simulink model "FFT_acquisition"  (R2022a)
settings: Solver=VariableStepAuto  StartTime=0.0  StopTime=0.001  RelTol=1e-3
values from neighbouring files (symbols this model uses):
  v = 2.5    [test.m]    (also in test_Datacode.m = 5)
undefined symbols (not defined in the file or in its folder): fdesignblkfcn, gcbh
libraries: simulink x3, dspxfrm3 x3, commchan3 x1, dsparch4 x1, dspfdesign x1, commrandsrc3 x1
settings Model: Creator=sky 2020  LastModifiedBy=sky 2020

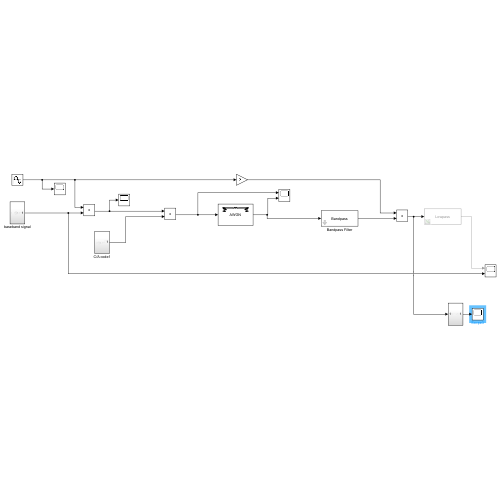
[thumbnail: Simulink's stored preview of the top-level diagram]
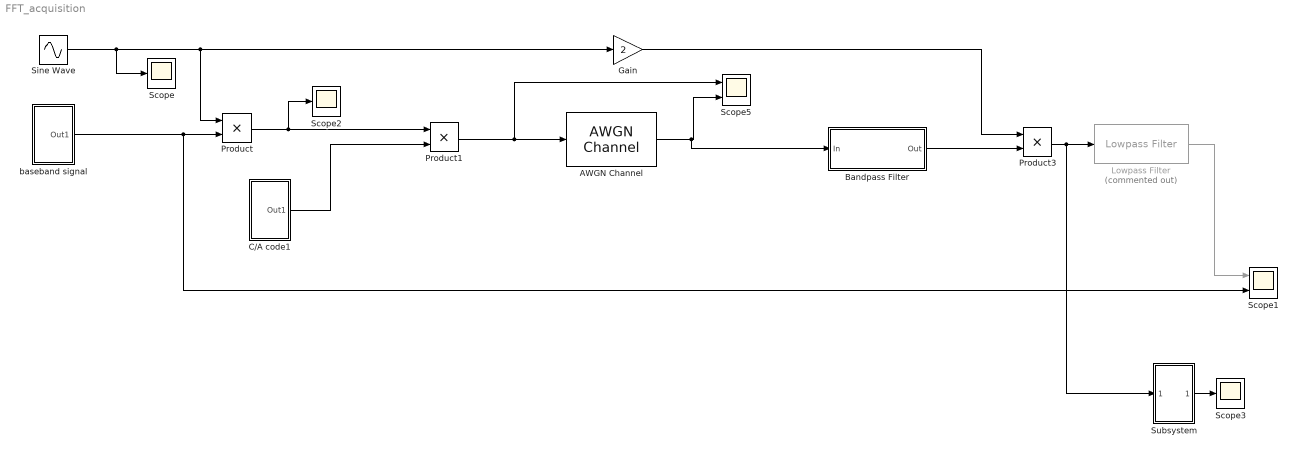
== system FFT_acquisition ==
  AWGN Channel : commchan3/AWGN Channel  InputProcessing=Columns as channels (frame based)  seed=67  noiseMode="Signal to noise ratio  (SNR)"  EbNodB=0  EsNodB=10  SNRdB=0  bitsPerSym=1  Ps=1  Tsym=1  variance=1
  Bandpass Filter : Subsystem  DialogController=fdesignblkfcn  InitFcn=fdesignblkfcn(gcbh, {'InitFcn'});  mask(Bandpass Filter){}
      mask help: Design a bandpass filter
      settings: CopyFcn=fdesignblkfcn(gcbh, {'CopyFcn'});
      mask Help: helpview(mapfilelocation('dsp'), 'dspbandpassfilter');
      mask Display: disp('Bandpass');
  C/A code1 : Subsystem
  Gain : Gain  Gain=2
  Lowpass Filter : dspfdesign/Lowpass Filter  Commented=on  FilterType=FIR  DesignForMinimumOrder=on  FilterOrder=50  PassbandFrequency=1.2e3  StopbandFrequency=2e3  PassbandRipple=0.1  StopbandAttenuation=60  InheritSampleRate=off  SampleRate=157.742e2  SimulateUsing=Interpreted execution  roundingMode=Floor  coeffsDataTypeStr=fixdt(1,16)
  Product : Product
  Product1 : Product
  Product3 : Product
  Scope : Scope
  Scope1 : Scope  NumInputPorts=2
  Scope2 : Scope
  Scope3 : Scope
  Scope5 : Scope  NumInputPorts=2
  Sine Wave : Sin  Frequency=2*pi*157.542e6  Phase=pi/2  SampleTime=1/(v*157.542e6)
  Subsystem : Subsystem
  baseband signal : Subsystem
  wires:
  Sine Wave/1 -> Scope/1, Gain/1, Product/1
  AWGN Channel/1 -> Bandpass Filter/1(In), Scope5/2
  Lowpass Filter/1 -> Scope1/1
  Bandpass Filter/1(Out) -> Product3/2
  Product1/1 -> Scope5/1, AWGN Channel/1
  baseband signal/1(Out1) -> Scope1/2, Product/2
  C/A code1/1(Out1) -> Product1/2
  Gain/1 -> Product3/1
  Product/1 -> Scope2/1, Product1/1
  Product3/1 -> Subsystem/1(In1), Lowpass Filter/1
  Subsystem/1(Out1) -> Scope3/1

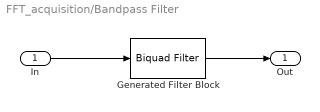
== system FFT_acquisition/Bandpass Filter ==
  In : Inport
  Generated Filter Block : dsparch4/Biquad Filter  Tag=BlockMethodSubSystem  FilterSource=Dialog parameters  CoeffSource=Specify via dialog  FilterObject=BQF  IIRFiltStruct=Direct form II  BiQuadCoeffs=[0.00380302990539071279 0 -0.00380302990539071279 1 1.61904346999335025 0.998458791755205466;0.00222628283797649028 0 -0.00222628283797649028 1 1.61451631506587345 0.998450612907040735;0.851459124863951367 0 -0.851459124863951367 1 1.61553762151329305 0.996911779330365899]  ScaleValues=[0.000919689030413472098;1;1;1]  IC=0  ICnum=0  ICden=0  a0Flag=Warning  optimizeScaleValues=off  ScaleValueMode=Specify via input port (g)  InputProcessing=Columns as channels (frame based)  roundingMode=Floor  overflowMode=off  scaleValueFracLength=14  denProdOutputFracLength=30  denAccumFracLength=30  secondMemoryFracLength=15
  Out : Outport  VectorParamsAs1DForOutWhenUnconnected=off
  wires:
  In/1 -> Generated Filter Block/1
  Generated Filter Block/1 -> Out/1

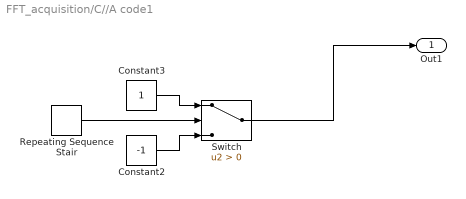
== system FFT_acquisition/C//A code1 ==
  Constant2 : Constant  Value=-1
  Constant3 : Constant
  Repeating Sequence Stair : simulink/Sources/Repeating Sequence Stair  OutValues=ca1  tsamp=1e-3/1023  OutMin=[]  OutMax=[]  OutDataTypeStr=double  OutputDataTypeScalingMode=double  OutDataType=fixdt(0,8)  ConRadixGroup=Best Precision: Vector-wise  OutScaling=2^-12
  Switch : Switch  Criteria=u2 > Threshold  SaturateOnIntegerOverflow=off  InputSameDT=off
  Out1 : Outport
  wires:
  Repeating Sequence Stair/1 -> Switch/2
  Constant2/1 -> Switch/3
  Constant3/1 -> Switch/1
  Switch/1 -> Out1/1

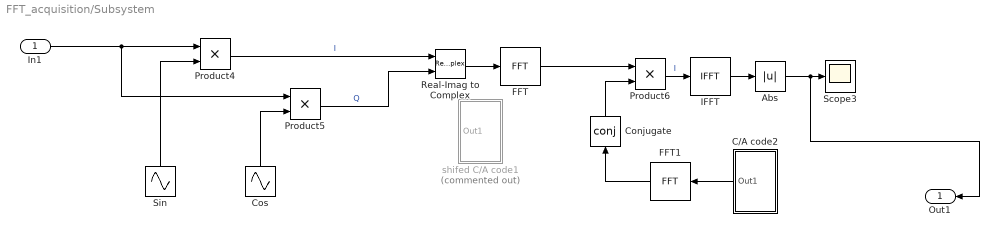
== system FFT_acquisition/Subsystem ==
  In1 : Inport
  Abs : Abs  SaturateOnIntegerOverflow=off
  C/A code2 : Subsystem
  Conjugate : Math  Operator=conj  SignedPower=on  RndMeth=Zero
  Cos : Sin  Frequency=2*pi*157.542e6  Phase=pi/2  SampleTime=1/(v*157.542e6)
  FFT : dspxfrm3/FFT  FFTImplementation=Auto  CompMethod=Table lookup  TableOpt=NEW  TableOptActive=Speed  BitRevOrder=off  Normalize=off  InheritFFTLength=on  FFTLength=64  WrapInput=on  roundingMode=Floor  overflowMode=off  firstCoeffDataTypeStr=Inherit: Same word length as input  firstCoeffLastDataTypeStr=Inherit: Same word length as input  outputMin=[]  outputMax=[]
  FFT1 : dspxfrm3/FFT  FFTImplementation=Auto  CompMethod=Table lookup  TableOpt=NEW  TableOptActive=Speed  BitRevOrder=off  Normalize=off  InheritFFTLength=on  FFTLength=64  WrapInput=on  roundingMode=Floor  overflowMode=off  firstCoeffDataTypeStr=Inherit: Same word length as input  firstCoeffLastDataTypeStr=Inherit: Same word length as input  outputMin=[]  outputMax=[]
  IFFT : dspxfrm3/IFFT  FFTImplementation=Auto  CompMethod=Table lookup  TableOpt=NEW  TableOptActive=Speed  BitRevOrder=off  cs_in=off  Normalize=on  InheritFFTLength=on  FFTLength=64  WrapInput=on  mode=Complex  outSamplingMode=Sample based  roundingMode=Floor  overflowMode=off  firstCoeffDataTypeStr=Inherit: Same word length as input  firstCoeffLastDataTypeStr=Inherit: Same word length as input  outputMin=[]  outputMax=[]
  Product4 : Product
  Product5 : Product
  Product6 : Product
  Real-Imag to Complex : RealImagToComplex
  Scope3 : Scope
  Sin : Sin  Frequency=2*pi*157.542e6  SampleTime=1/(v*157.542e6)
  shifed C/A code1 : Subsystem  Commented=on
  Out1 : Outport
  wires:
  Real-Imag to Complex/1 -> FFT/1
  Product5/1 -> Real-Imag to Complex/2  "Q"
  Sin/1 -> Product4/2
  Abs/1 -> Out1/1, Scope3/1
  Product4/1 -> Real-Imag to Complex/1  "I"
  IFFT/1 -> Abs/1
  Cos/1 -> Product5/2
  FFT1/1 -> Conjugate/1
  C/A code2/1(Out1) -> FFT1/1
  Conjugate/1 -> Product6/2
  Product6/1 -> IFFT/1  "I"
  FFT/1 -> Product6/1
  In1/1 -> Product5/1, Product4/1

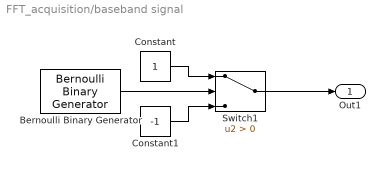
== system FFT_acquisition/baseband signal ==
  Bernoulli Binary Generator : commrandsrc3/Bernoulli Binary Generator  ProbabilityOfZero=0.5  SeedSource=Auto  Seed=0  SampleTime=1/1e3  SamplesPerFrame=1  OutputDataType=double  SimulateUsing=Interpreted execution
  Constant : Constant
  Constant1 : Constant  Value=-1
  Switch1 : Switch  Criteria=u2 > Threshold  SaturateOnIntegerOverflow=off  InputSameDT=off
  Out1 : Outport
  wires:
  Constant1/1 -> Switch1/3
  Constant/1 -> Switch1/1
  Bernoulli Binary Generator/1 -> Switch1/2
  Switch1/1 -> Out1/1

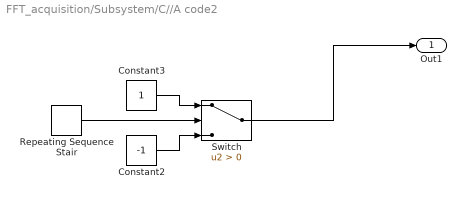
== system FFT_acquisition/Subsystem/C//A code2 ==
  Constant2 : Constant  Value=-1
  Constant3 : Constant
  Repeating Sequence Stair : simulink/Sources/Repeating Sequence Stair  OutValues=ca1  tsamp=1e-3/1023  OutMin=[]  OutMax=[]  OutDataTypeStr=double  OutputDataTypeScalingMode=double  OutDataType=fixdt(0,8)  ConRadixGroup=Best Precision: Vector-wise  OutScaling=2^-12
  Switch : Switch  Criteria=u2 > Threshold  SaturateOnIntegerOverflow=off  InputSameDT=off
  Out1 : Outport
  wires:
  Repeating Sequence Stair/1 -> Switch/2
  Constant2/1 -> Switch/3
  Constant3/1 -> Switch/1
  Switch/1 -> Out1/1

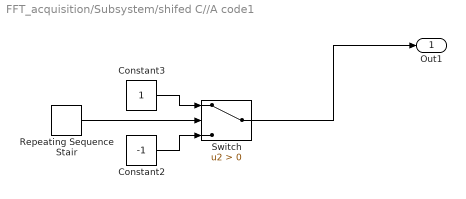
== system FFT_acquisition/Subsystem/shifed C//A code1 ==
  Constant2 : Constant  Value=-1
  Constant3 : Constant
  Repeating Sequence Stair : simulink/Sources/Repeating Sequence Stair  OutValues=ca1  tsamp=1e-3/1023  OutMin=[]  OutMax=[]  OutDataTypeStr=double  OutputDataTypeScalingMode=double  OutDataType=fixdt(0,8)  ConRadixGroup=Best Precision: Vector-wise  OutScaling=2^-12
  Switch : Switch  Criteria=u2 > Threshold  SaturateOnIntegerOverflow=off  InputSameDT=off
  Out1 : Outport
  wires:
  Repeating Sequence Stair/1 -> Switch/2
  Constant2/1 -> Switch/3
  Constant3/1 -> Switch/1
  Switch/1 -> Out1/1
